simulink model "Part2FullModel"  (R2017a)
settings: Solver=VariableStepAuto  StartTime=0.0  StopTime=1000  RelTol=1e-3
values from neighbouring files (symbols this model uses):
  A = [-0.322, 0.052, 0.028, -1.12, 0.002 ... (first row only)    [InitialisePart1.m]
  a_phi_1 = 2.87    [InitialisePart1.m]    (also in init.m)
  a_phi_2 = -0.65    [InitialisePart1.m]    (also in init.m)
  B = [0; 0; 0; 0; -7.5]    [InitialisePart1.m]
  d = 1.5*deg2rad    (= 0.0261799387799)    [InitialisePart1.m]    (also in init.m)
  g = 9.81    [InitialisePart1.m]    (also in init.m = -9.81)
  k_d_phi = (2*zeta*omega_n-a_phi_1)/a_phi_2    [InitialisePart1.m]    (also in init.m)
  k_i_khi = (V_g/g)*(omega_x)^2    [InitialisePart1.m]    (also in init.m)
  k_i_phi = -1    [InitialisePart1.m]    (also in init.m = 1)
  k_p_khi = (V_g/g)*2*zeta_x*omega_x    [InitialisePart1.m]    (also in init.m)
  k_p_phi = delta_a_max/e_max*sign(a_phi_2)    [InitialisePart1.m]    (also in init.m)
  V_g = V_a    (= 161.111111111)    [InitialisePart1.m]    (also in init.m)
undefined symbols (not defined in the file or in its folder): C
settings Model: Creator=martimos  LastModifiedBy=Ambjørn

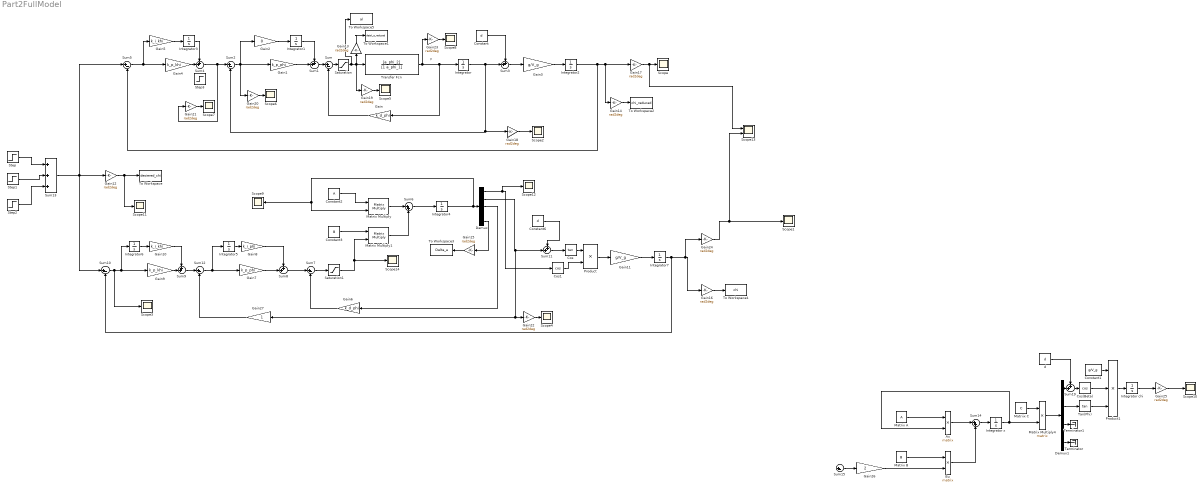
== system Part2FullModel ==
  note: p
  Ax : Product  Multiplication=Matrix(*)
  Bu : Product  Multiplication=Matrix(*)
  Constant : Constant  Value=d
  Constant1 : Constant  Value=g/V_g
  Constant2 : Constant  Value=A
  Constant3 : Constant  Value=B
  Constant6 : Constant  Value=d
  Cos : Trigonometry  Operator=tan
  Cos(Beta) : Trigonometry  Operator=cos
  Cos1 : Trigonometry  Operator=cos
  Demux : Demux  Outputs=5
  Demux1 : Demux
  Gain : Gain  Gain=k_d_phi
  Gain1 : Gain  Gain=k_p_phi
  Gain10 : Gain  Gain=k_i_khi
  Gain11 : Gain  Gain=g/V_g
  Gain{12..25} (14 alike) : Gain  Gain=rad2deg
  Gain2 : Gain  Gain=0
  Gain26 : Gain  Gain=2
  Gain27 : Gain
  Gain3 : Gain  Gain=g/V_g
  Gain4 : Gain  Gain=k_p_khi
  Gain5 : Gain  Gain=k_i_khi
  Gain6 : Gain  Gain=k_d_phi
  Gain7 : Gain  Gain=k_p_phi
  Gain8 : Gain  Gain=k_i_phi
  Gain9 : Gain  Gain=k_p_khi
  Integrator{,1..7} (8 alike) : Integrator
  "Integrator chi " : Integrator
  "Integrator x " : Integrator
  Matriix C : Constant  Value=C
  Matrix A : Constant  Value=A
  Matrix B : Constant  Value=B
  Matrix Multiply : Product  Multiplication=Matrix(*)
  Matrix Multiply1 : Product  Multiplication=Matrix(*)
  Matrix Multiply4 : Product  Multiplication=Matrix(*)
  Product : Product
  Product1 : Product  Inputs=3
  Saturation : Saturate  UpperLimit=30*deg2rad  LowerLimit=-30*deg2rad
  Saturation1 : Saturate  UpperLimit=0.523333  LowerLimit=-0.52333
  Scope{,1..12,14} (14 alike) : Scope
  Scope13 : Scope  NumInputPorts=2
  Step : Step  Time=5  After=2*deg2rad  SampleTime=0
  Step1 : Step  Time=50  After=-2*deg2rad  SampleTime=0
  Step2 : Step  Time=150  After=-4*deg2rad  SampleTime=0
  Step3 : Step  Time=5  After=15*deg2rad  SampleTime=0
  Sum{,2,5,7,10,12,15} (7 alike) : Sum  Inputs=|+-
  Sum{1,3..4,8..9,11,19} (7 alike) : Sum  Inputs=++|
  Sum13 : Sum  Inputs=+++
  Sum14 : Sum  Inputs=|++
  Sum6 : Sum  Inputs=|++
  Tan(Phi) : Trigonometry  Operator=tan
  Terminator : Terminator
  Terminator1 : Terminator
  To Workspace : ToWorkspace  VariableName=desiered_chi  SaveFormat=Timeseries  SampleTime=-1
  To Workspace1 : ToWorkspace  VariableName=detal_a_reduced  SaveFormat=Timeseries  SampleTime=-1
  To Workspace2 : ToWorkspace  VariableName=chi_reduced  SaveFormat=Timeseries  SampleTime=-1
  To Workspace3 : ToWorkspace  VariableName=Delta_a  SaveFormat=Timeseries  SampleTime=-1
  To Workspace4 : ToWorkspace  VariableName=chi  SaveFormat=Timeseries  SampleTime=-1
  To Workspace5 : ToWorkspace  VariableName=al  SaveFormat=Timeseries  SampleTime=-1
  Transfer Fcn : TransferFcn  Numerator=[a_phi_2]  Denominator=[1 a_phi_1]
  d : Constant  Value=d
  wires:
  Transfer Fcn/1 -> Gain23/1, Gain/1, Integrator/1
  Sum/1 -> Saturation/1
  Gain/1 -> Sum/2
  Sum1/1 -> Sum/1
  Gain1/1 -> Sum1/2
  Sum2/1 -> Gain2/1, Gain20/1, Gain1/1
  Integrator/1 -> Sum3/2, Sum2/2, Gain18/1
  Sum3/1 -> Gain3/1
  Constant/1 -> Sum3/1
  Gain3/1 -> Integrator2/1
  Integrator2/1 -> Sum5/2, Gain14/1, Gain17/1
  Gain4/1 -> Sum4/2
  Sum5/1 -> Gain5/1, Gain4/1
  Sum6/1 -> Integrator4/1
  Constant2/1 -> Matrix Multiply/1
  Matrix Multiply/1 -> Sum6/1
  Matrix Multiply1/1 -> Sum6/2
  Constant3/1 -> Matrix Multiply1/1
  Integrator4/1 -> Demux/1, Scope9/1, Matrix Multiply/2
  Gain7/1 -> Sum8/2
  Sum8/1 -> Sum7/1
  Integrator5/1 -> Gain8/1
  Gain8/1 -> Sum8/1
  Gain6/1 -> Sum7/2
  Sum10/1 -> Scope3/1, Integrator6/1, Gain9/1
  Gain10/1 -> Sum9/1
  Gain9/1 -> Sum9/2
  Sum13/1 -> Sum10/1, Sum5/1, Gain12/1
  Constant6/1 -> Sum11/1
  Demux/2 -> Gain27/1, Gain22/1, Sum11/2
  Integrator7/1 -> Sum10/2, Gain16/1, Gain24/1
  Sum11/1 -> Cos/1
  Gain11/1 -> Integrator7/1
  Integrator6/1 -> Gain10/1
  Product/1 -> Gain11/1
  Cos/1 -> Product/1
  Cos1/1 -> Product/2
  Sum7/1 -> Saturation1/1
  Sum9/1 -> Sum12/1
  Sum12/1 -> Integrator5/1, Gain7/1
  Step/1 -> Sum13/1
  Step1/1 -> Sum13/2
  Step2/1 -> Sum13/3
  Gain12/1 -> Scope11/1, To Workspace/1
  Gain13/1 -> To Workspace1/1
  Gain14/1 -> To Workspace2/1
  Demux/5 -> Gain15/1
  Gain15/1 -> To Workspace3/1
  Gain16/1 -> To Workspace4/1
  Gain17/1 -> Scope13/1, Scope/1
  Gain18/1 -> Scope2/1
  Saturation/1 -> To Workspace5/1, Gain19/1, Gain13/1, Transfer Fcn/1
  Gain19/1 -> Scope5/1
  Gain20/1 -> Scope6/1
  Gain21/1 -> Scope7/1
  Gain22/1 -> Scope4/1
  Gain23/1 -> Scope8/1
  Sum4/1 -> Gain21/1, Sum2/1
  Gain24/1 -> Scope13/2, Scope1/1
  Matrix A/1 -> Ax/1
  Matrix B/1 -> Bu/1
  Ax/1 -> Sum14/1
  Bu/1 -> Sum14/2
  Sum14/1 -> "Integrator x "/1
  "Integrator x "/1 -> Ax/2, Matrix Multiply4/2
  Matriix C/1 -> Matrix Multiply4/1
  Gain25/1 -> Scope10/1
  Matrix Multiply4/1 -> Demux1/1
  Demux1/4 -> Terminator/1
  Constant1/1 -> Product1/1
  Demux1/2 -> Tan(Phi)/1
  Cos(Beta)/1 -> Product1/2
  Tan(Phi)/1 -> Product1/3
  Product1/1 -> "Integrator chi "/1
  "Integrator chi "/1 -> Gain25/1
  Sum19/1 -> Cos(Beta)/1
  d/1 -> Sum19/1
  Gain5/1 -> Integrator3/1
  Integrator3/1 -> Sum4/1
  Gain2/1 -> Integrator1/1
  Integrator1/1 -> Sum1/1
  Sum15/1 -> Gain26/1
  Demux1/3 -> Terminator1/1
  Gain26/1 -> Bu/2
  Demux1/1 -> Sum19/2
  Gain27/1 -> Sum12/2
  Demux/1 -> Scope12/1, Cos1/1
  Demux/3 -> Gain6/1
  Saturation1/1 -> Scope14/1, Matrix Multiply1/2
